simulink model "stm32f4_rtc_configure_demo"  (Simulink 7.3)
settings: Solver=FixedStepDiscrete  SolverMode=SingleTasking  StartTime=0.0  StopTime=10.0  RelTol=1e-3
PreLoadFcn:
  | waijung.modelPreload; % Required for working with Waijung Blockset. Do not remove.
undefined symbols (not defined in the file): HSEOSC, Link, LQFP176, ST, STM32F417IG
libraries: simulink x54, amg_high_precision_rtc x5, stm32f4_io_lib x2, stm32f4_device_config_lib x1
(part 2 of 3)

== system stm32f4_rtc_configure_demo/Display Date/Time/Display Second ==
  In1 : Inport
  In2 : Inport  Port=2
  In3 : Inport  Port=3
  Data Type Conversion : DataTypeConversion  OutDataTypeMode=uint8  OutDataType=fixdt(1, 16)  OutScaling=2^0  OutDataTypeStr=uint8
  Logical Operator : Logic  Inputs=3  AllPortsSameDT=off  OutDataTypeMode=boolean  LogicDataType=fixdt(0, 8)  OutDataTypeStr=boolean
  Switch : Switch  Criteria=u2 ~= 0  OutDataType=fixdt(1, 16)  OutScaling=2^0
  Volatile Data Storage Read : S-Function  FunctionName=waijung_vdata_read  Parameters=storagename,varname,sampletime,sampletimestr,blockid,storagetype,storagetypestr  EnableBusSupport=off  mask(waijung_vdata_read){storagename=str_blank2, varname=CharacterLCDSetupVolatileDataStorage7_str_blank2, sampletime=inf, sampletimestr=0.01, blockid=DisplayDateTimeDisplaySecondVolatileDataStorageRead, storagetype=string, storagetypestr=uint32_t}
      mask prompts: storagename "Storage Name"; varname "Variable name"; sampletime "Sample time (sec)"; sampletimestr "Compiled sample time (sec) in string"; storagetype "Data type"; storagetypestr "Data type string"
      mask help: This block implements read data from a buffer.
      mask init:
      | waijung_vdata_read_callback('init');
      mask Help: web(fullfile(waijungdocroot,'waijung_vdata_read.htm'))
      mask StyleString: popup(str_date|str_month|str_year|str_hour|str_minute|str_second|str_blank2|LCD_Buffer),edit,edit,edit,edit,edit,edit
      mask CallbackString: waijung_vdata_read_callback('storagename');|waijung_vdata_read_callback('varname');|waijung_vdata_read_callback('sampletime');|waijung_vdata_read_callback('sampletimestr');|waijung_vdata_read_callback('blockid');|waijung_vdata_read_callback('storagetype');|
      mask Display: text(0.05, 0.5, 'Buffer: str_blank2','ver','middle','hor','left');port_label('output',1,'D1(string)')
  Volatile Data Storage Read1 : S-Function  FunctionName=waijung_vdata_read  Parameters=storagename,varname,sampletime,sampletimestr,blockid,storagetype,storagetypestr  EnableBusSupport=off  mask(waijung_vdata_read){storagename=str_second, varname=CharacterLCDSetupVolatileDataStorage6_str_second, sampletime=inf, sampletimestr=0.01, blockid=DisplayDateTimeDisplaySecondVolatileDataStorageRead1, storagetype=string, storagetypestr=uint32_t}
      mask prompts: storagename "Storage Name"; varname "Variable name"; sampletime "Sample time (sec)"; sampletimestr "Compiled sample time (sec) in string"; storagetype "Data type"; storagetypestr "Data type string"
      mask help: This block implements read data from a buffer.
      mask init:
      | waijung_vdata_read_callback('init');
      mask Help: web(fullfile(waijungdocroot,'waijung_vdata_read.htm'))
      mask StyleString: popup(str_date|str_month|str_year|str_hour|str_minute|str_second|str_blank2|LCD_Buffer),edit,edit,edit,edit,edit,edit
      mask CallbackString: waijung_vdata_read_callback('storagename');|waijung_vdata_read_callback('varname');|waijung_vdata_read_callback('sampletime');|waijung_vdata_read_callback('sampletimestr');|waijung_vdata_read_callback('blockid');|waijung_vdata_read_callback('storagetype');|
      mask Display: text(0.05, 0.5, 'Buffer: str_second','ver','middle','hor','left');port_label('output',1,'D1(string)')
  Out1 : Outport
  wires:
  In3/1 -> Logical Operator/3
  Switch/1 -> Out1/1
  In2/1 -> Logical Operator/2
  In1/1 -> Logical Operator/1
  Volatile Data Storage Read1/1 -> Switch/3
  Volatile Data Storage Read/1 -> Switch/1
  Logical Operator/1 -> Data Type Conversion/1
  Data Type Conversion/1 -> Switch/2

== system stm32f4_rtc_configure_demo/Display Date/Time/Display Year ==
  In1 : Inport
  In2 : Inport  Port=2
  In3 : Inport  Port=3
  Data Type Conversion : DataTypeConversion  OutDataTypeMode=uint8  OutDataType=fixdt(1, 16)  OutScaling=2^0  OutDataTypeStr=uint8
  Logical Operator : Logic  Inputs=3  AllPortsSameDT=off  OutDataTypeMode=boolean  LogicDataType=fixdt(0, 8)  OutDataTypeStr=boolean
  Switch : Switch  Criteria=u2 ~= 0  OutDataType=fixdt(1, 16)  OutScaling=2^0
  Volatile Data Storage Read : S-Function  FunctionName=waijung_vdata_read  Parameters=storagename,varname,sampletime,sampletimestr,blockid,storagetype,storagetypestr  EnableBusSupport=off  mask(waijung_vdata_read){storagename=str_blank2, varname=CharacterLCDSetupVolatileDataStorage7_str_blank2, sampletime=inf, sampletimestr=0.01, blockid=DisplayDateTimeDisplayYearVolatileDataStorageRead, storagetype=string, storagetypestr=uint32_t}
      mask prompts: storagename "Storage Name"; varname "Variable name"; sampletime "Sample time (sec)"; sampletimestr "Compiled sample time (sec) in string"; storagetype "Data type"; storagetypestr "Data type string"
      mask help: This block implements read data from a buffer.
      mask init:
      | waijung_vdata_read_callback('init');
      mask Help: web(fullfile(waijungdocroot,'waijung_vdata_read.htm'))
      mask StyleString: popup(str_date|str_month|str_year|str_hour|str_minute|str_second|str_blank2|LCD_Buffer),edit,edit,edit,edit,edit,edit
      mask CallbackString: waijung_vdata_read_callback('storagename');|waijung_vdata_read_callback('varname');|waijung_vdata_read_callback('sampletime');|waijung_vdata_read_callback('sampletimestr');|waijung_vdata_read_callback('blockid');|waijung_vdata_read_callback('storagetype');|
      mask Display: text(0.05, 0.5, 'Buffer: str_blank2','ver','middle','hor','left');port_label('output',1,'D1(string)')
  Volatile Data Storage Read1 : S-Function  FunctionName=waijung_vdata_read  Parameters=storagename,varname,sampletime,sampletimestr,blockid,storagetype,storagetypestr  EnableBusSupport=off  mask(waijung_vdata_read){storagename=str_year, varname=CharacterLCDSetupVolatileDataStorage3_str_year, sampletime=inf, sampletimestr=0.01, blockid=DisplayDateTimeDisplayYearVolatileDataStorageRead1, storagetype=string, storagetypestr=uint32_t}
      mask prompts: storagename "Storage Name"; varname "Variable name"; sampletime "Sample time (sec)"; sampletimestr "Compiled sample time (sec) in string"; storagetype "Data type"; storagetypestr "Data type string"
      mask help: This block implements read data from a buffer.
      mask init:
      | waijung_vdata_read_callback('init');
      mask Help: web(fullfile(waijungdocroot,'waijung_vdata_read.htm'))
      mask StyleString: popup(str_date|str_month|str_year|str_hour|str_minute|str_second|str_blank2|LCD_Buffer),edit,edit,edit,edit,edit,edit
      mask CallbackString: waijung_vdata_read_callback('storagename');|waijung_vdata_read_callback('varname');|waijung_vdata_read_callback('sampletime');|waijung_vdata_read_callback('sampletimestr');|waijung_vdata_read_callback('blockid');|waijung_vdata_read_callback('storagetype');|
      mask Display: text(0.05, 0.5, 'Buffer: str_year','ver','middle','hor','left');port_label('output',1,'D1(string)')
  Out1 : Outport
  wires:
  Data Type Conversion/1 -> Switch/2
  Logical Operator/1 -> Data Type Conversion/1
  Volatile Data Storage Read/1 -> Switch/1
  Volatile Data Storage Read1/1 -> Switch/3
  In1/1 -> Logical Operator/1
  In2/1 -> Logical Operator/2
  Switch/1 -> Out1/1
  In3/1 -> Logical Operator/3

== system stm32f4_rtc_configure_demo/Display Date/Time/Get Date as String ==
  Printf1 : S-Function  FunctionName=waijung_printf  Parameters=storagename,printfformat,formatcode,varname,sampletime,sampletimestr,blockid  EnableBusSupport=off  mask(waijung_printf){storagename=str_date, printfformat=%2u/, formatcode=u, varname=CharacterLCDSetupVolatileDataStorage1_str_date, sampletime=-1, sampletimestr=0.01, blockid=DisplayDateTimeGetDateasStringPrintf1}
      mask prompts: storagename "Storage Name"; printfformat "Printf format"; formatcode "Printf format code"; varname "Variable name"; sampletime "Sample time (sec)"; sampletimestr "Compiled sample time (sec) in string"
      mask help: This block implements printf command.
      mask init:
      | waijung_printf_callback('init');
      mask Help: web(fullfile(waijungdocroot,'waijung_printf.htm'))
      mask StyleString: popup(str_date|str_month|str_year|str_hour|str_minute|str_second|str_blank2|LCD_Buffer),edit,edit,edit,edit,edit,edit
      mask CallbackString: waijung_printf_callback('storagename');|waijung_printf_callback('printfformat');|waijung_printf_callback('formatcode');|waijung_printf_callback('varname');|waijung_printf_callback('sampletime');|waijung_printf_callback('sampletimestr');|waijung_printf_callback('blockid');
      mask Display: text(0.95, 0.5, 'Buffer: str_date\nTs (sec): 0.01','ver','middle','hor','right');port_label('input',1,'D1(%u)');
  Printf2 : S-Function  FunctionName=waijung_printf  Parameters=storagename,printfformat,formatcode,varname,sampletime,sampletimestr,blockid  EnableBusSupport=off  mask(waijung_printf){storagename=str_month, printfformat=%2u/, formatcode=u, varname=CharacterLCDSetupVolatileDataStorage2_str_month, sampletime=-1, sampletimestr=0.01, blockid=DisplayDateTimeGetDateasStringPrintf2}
      mask prompts: storagename "Storage Name"; printfformat "Printf format"; formatcode "Printf format code"; varname "Variable name"; sampletime "Sample time (sec)"; sampletimestr "Compiled sample time (sec) in string"
      mask help: This block implements printf command.
      mask init:
      | waijung_printf_callback('init');
      mask Help: web(fullfile(waijungdocroot,'waijung_printf.htm'))
      mask StyleString: popup(str_date|str_month|str_year|str_hour|str_minute|str_second|str_blank2|LCD_Buffer),edit,edit,edit,edit,edit,edit
      mask CallbackString: waijung_printf_callback('storagename');|waijung_printf_callback('printfformat');|waijung_printf_callback('formatcode');|waijung_printf_callback('varname');|waijung_printf_callback('sampletime');|waijung_printf_callback('sampletimestr');|waijung_printf_callback('blockid');
      mask Display: text(0.95, 0.5, 'Buffer: str_month\nTs (sec): 0.01','ver','middle','hor','right');port_label('input',1,'D1(%u)');
  Printf3 : S-Function  FunctionName=waijung_printf  Parameters=storagename,printfformat,formatcode,varname,sampletime,sampletimestr,blockid  EnableBusSupport=off  mask(waijung_printf){storagename=str_year, printfformat=%2u, formatcode=u, varname=CharacterLCDSetupVolatileDataStorage3_str_year, sampletime=-1, sampletimestr=0.01, blockid=DisplayDateTimeGetDateasStringPrintf3}
      mask prompts: storagename "Storage Name"; printfformat "Printf format"; formatcode "Printf format code"; varname "Variable name"; sampletime "Sample time (sec)"; sampletimestr "Compiled sample time (sec) in string"
      mask help: This block implements printf command.
      mask init:
      | waijung_printf_callback('init');
      mask Help: web(fullfile(waijungdocroot,'waijung_printf.htm'))
      mask StyleString: popup(str_date|str_month|str_year|str_hour|str_minute|str_second|str_blank2|LCD_Buffer),edit,edit,edit,edit,edit,edit
      mask CallbackString: waijung_printf_callback('storagename');|waijung_printf_callback('printfformat');|waijung_printf_callback('formatcode');|waijung_printf_callback('varname');|waijung_printf_callback('sampletime');|waijung_printf_callback('sampletimestr');|waijung_printf_callback('blockid');
      mask Display: text(0.95, 0.5, 'Buffer: str_year\nTs (sec): 0.01','ver','middle','hor','right');port_label('input',1,'D1(%u)');
  RTC Date Read : S-Function  FunctionName=stm32f4_rtc  Parameters=inputtypearray,outputtypearray,confstr,sampletime,sampletimestr,blockid  EnableBusSupport=off  mask(stm32f4_rtc){configuration=DateRead, clocksource=LSE (32.768kHz), dataformat=BIN, hourformat=HourFormat_24, inputtypearray=[0], outputtypearray=[4 3 3 3 3], confstr=["DateRead","LSE (32.768kHz)","BIN","HourFormat_24"], sampletime=0.01, sampletimestr=0.01, blockid=DisplayDateTimeGetDateasStringRTCDateRead}
      mask prompts: clocksource "Clock source"; dataformat "Format"; hourformat "Hour format"; inputtypearray "Input type array"; outputtypearray "Output type array"; confstr "Configuration string"; sampletime "Sample time (sec)"; sampletimestr "Compiled sample time (sec) in string"
      mask init:
      | stm32f4_rtc_callback('init');
      mask Help: web(fullfile(waijungdocroot,'stm32f4_rtc_setup.htm'), '-browser')
      mask StyleString: popup(Setup|DateRead|TimeRead|DateWrite|TimeWrite),popup(LSE (32.768kHz)|LSI),popup(BCD|BIN),popup(HourFormat_24|HourFormat_12),edit,edit,edit,edit,edit,edit
      mask CallbackString: stm32f4_rtc_callback('configuration');||stm32f4_rtc_callback('dataformat');||||stm32f4_rtc_callback('confstr');|stm32f4_rtc_callback('sampletime');|stm32f4_rtc_callback('sampletimestr');|stm32f4_rtc_callback('blockid');
      mask Display: text(0.05, 0.5, 'Module: RTC (DateRead)\nFormat: BIN\nTs (sec): 0.01','ver','middle','hor','left');port_label('output', 1,'Day');port_label('output', 2,'Date');port_label('output', 3,'Month');port_label('output', 4,'Year');
  Terminator : Terminator
  wires:
  RTC Date Read/2 -> Printf1/1
  RTC Date Read/4 -> Printf3/1
  RTC Date Read/3 -> Printf2/1
  RTC Date Read/1 -> Terminator/1

== system stm32f4_rtc_configure_demo/Display Date/Time/Get Time as String ==
  Printf4 : S-Function  FunctionName=waijung_printf  Parameters=storagename,printfformat,formatcode,varname,sampletime,sampletimestr,blockid  EnableBusSupport=off  mask(waijung_printf){storagename=str_hour, printfformat=%2u:, formatcode=u, varname=CharacterLCDSetupVolatileDataStorage4_str_hour, sampletime=-1, sampletimestr=0.01, blockid=DisplayDateTimeGetTimeasStringPrintf4}
      mask prompts: storagename "Storage Name"; printfformat "Printf format"; formatcode "Printf format code"; varname "Variable name"; sampletime "Sample time (sec)"; sampletimestr "Compiled sample time (sec) in string"
      mask help: This block implements printf command.
      mask init:
      | waijung_printf_callback('init');
      mask Help: web(fullfile(waijungdocroot,'waijung_printf.htm'))
      mask StyleString: popup(str_date|str_month|str_year|str_hour|str_minute|str_second|str_blank2|LCD_Buffer),edit,edit,edit,edit,edit,edit
      mask CallbackString: waijung_printf_callback('storagename');|waijung_printf_callback('printfformat');|waijung_printf_callback('formatcode');|waijung_printf_callback('varname');|waijung_printf_callback('sampletime');|waijung_printf_callback('sampletimestr');|waijung_printf_callback('blockid');
      mask Display: text(0.95, 0.5, 'Buffer: str_hour\nTs (sec): 0.01','ver','middle','hor','right');port_label('input',1,'D1(%u)');
  Printf5 : S-Function  FunctionName=waijung_printf  Parameters=storagename,printfformat,formatcode,varname,sampletime,sampletimestr,blockid  EnableBusSupport=off  mask(waijung_printf){storagename=str_minute, printfformat=%2u:, formatcode=u, varname=CharacterLCDSetupVolatileDataStorage5_str_minute, sampletime=-1, sampletimestr=0.01, blockid=DisplayDateTimeGetTimeasStringPrintf5}
      mask prompts: storagename "Storage Name"; printfformat "Printf format"; formatcode "Printf format code"; varname "Variable name"; sampletime "Sample time (sec)"; sampletimestr "Compiled sample time (sec) in string"
      mask help: This block implements printf command.
      mask init:
      | waijung_printf_callback('init');
      mask Help: web(fullfile(waijungdocroot,'waijung_printf.htm'))
      mask StyleString: popup(str_date|str_month|str_year|str_hour|str_minute|str_second|str_blank2|LCD_Buffer),edit,edit,edit,edit,edit,edit
      mask CallbackString: waijung_printf_callback('storagename');|waijung_printf_callback('printfformat');|waijung_printf_callback('formatcode');|waijung_printf_callback('varname');|waijung_printf_callback('sampletime');|waijung_printf_callback('sampletimestr');|waijung_printf_callback('blockid');
      mask Display: text(0.95, 0.5, 'Buffer: str_minute\nTs (sec): 0.01','ver','middle','hor','right');port_label('input',1,'D1(%u)');
  Printf6 : S-Function  FunctionName=waijung_printf  Parameters=storagename,printfformat,formatcode,varname,sampletime,sampletimestr,blockid  EnableBusSupport=off  mask(waijung_printf){storagename=str_second, printfformat=%2u, formatcode=u, varname=CharacterLCDSetupVolatileDataStorage6_str_second, sampletime=-1, sampletimestr=0.01, blockid=DisplayDateTimeGetTimeasStringPrintf6}
      mask prompts: storagename "Storage Name"; printfformat "Printf format"; formatcode "Printf format code"; varname "Variable name"; sampletime "Sample time (sec)"; sampletimestr "Compiled sample time (sec) in string"
      mask help: This block implements printf command.
      mask init:
      | waijung_printf_callback('init');
      mask Help: web(fullfile(waijungdocroot,'waijung_printf.htm'))
      mask StyleString: popup(str_date|str_month|str_year|str_hour|str_minute|str_second|str_blank2|LCD_Buffer),edit,edit,edit,edit,edit,edit
      mask CallbackString: waijung_printf_callback('storagename');|waijung_printf_callback('printfformat');|waijung_printf_callback('formatcode');|waijung_printf_callback('varname');|waijung_printf_callback('sampletime');|waijung_printf_callback('sampletimestr');|waijung_printf_callback('blockid');
      mask Display: text(0.95, 0.5, 'Buffer: str_second\nTs (sec): 0.01','ver','middle','hor','right');port_label('input',1,'D1(%u)');
  RTC Time Read : S-Function  FunctionName=stm32f4_rtc  Parameters=inputtypearray,outputtypearray,confstr,sampletime,sampletimestr,blockid  EnableBusSupport=off  mask(stm32f4_rtc){configuration=TimeRead, clocksource=LSE (32.768kHz), dataformat=BIN, hourformat=HourFormat_24, inputtypearray=[0], outputtypearray=[3 3 3 3], confstr=["TimeRead","LSE (32.768kHz)","BIN","HourFormat_24"], sampletime=0.01, sampletimestr=0.01, blockid=DisplayDateTimeGetTimeasStringRTCTimeRead}
      mask prompts: clocksource "Clock source"; dataformat "Format"; hourformat "Hour format"; inputtypearray "Input type array"; outputtypearray "Output type array"; confstr "Configuration string"; sampletime "Sample time (sec)"; sampletimestr "Compiled sample time (sec) in string"
      mask init:
      | stm32f4_rtc_callback('init');
      mask Help: web(fullfile(waijungdocroot,'stm32f4_rtc_setup.htm'), '-browser')
      mask StyleString: popup(Setup|DateRead|TimeRead|DateWrite|TimeWrite),popup(LSE (32.768kHz)|LSI),popup(BCD|BIN),popup(HourFormat_24|HourFormat_12),edit,edit,edit,edit,edit,edit
      mask CallbackString: stm32f4_rtc_callback('configuration');||stm32f4_rtc_callback('dataformat');||||stm32f4_rtc_callback('confstr');|stm32f4_rtc_callback('sampletime');|stm32f4_rtc_callback('sampletimestr');|stm32f4_rtc_callback('blockid');
      mask Display: text(0.05, 0.5, 'Module: RTC (TimeRead)\nFormat: BIN\nTs (sec): 0.01','ver','middle','hor','left');port_label('output', 1,'Hour');port_label('output', 2,'Minute');port_label('output', 3,'Second');
  wires:
  RTC Time Read/3 -> Printf6/1
  RTC Time Read/2 -> Printf5/1
  RTC Time Read/1 -> Printf4/1

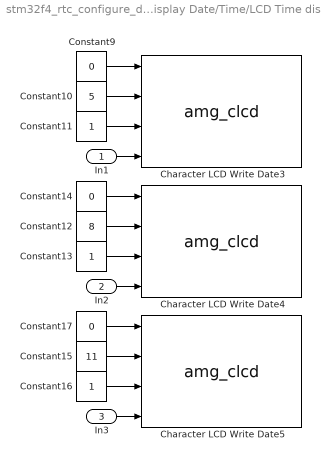
== system stm32f4_rtc_configure_demo/Display Date/Time/LCD Time display ==
  In1 : Inport
  In2 : Inport  Port=2
  In3 : Inport  Port=3
  Character LCD Write Date3 : S-Function  FunctionName=amg_clcd  Parameters=module,configuration,inputtypearray,outputtypearray,confstr,sampletime,sampletimestr,blockid  EnableBusSupport=off  mask(amg_clcd){configuration=Transaction, module=1, model=amg CLCD Std, interface=4-bits, linecount=4, columncount=20, gpiotype=Push-pull, controlport=E, control_rs=15, control_rw=13, control_en=11, dataport=A, data0=7, data1=5, data2=3, data3=1, usestringbuffer=off, stringbuffer=<empty>, varname=, inputtypearray=[4 -1 -1 -1 -1], outputtypearray=[0], confstr=["4","4","20","PP","E","15","11","13","","A","","","","","7","5","3","1","0","","1","0","0","0","1","0","0","0","0","stm32f4"], sampletime=-1, sampletimestr=0.01, blockid=DisplayDateTimeLCDTimedisplayCharacterLCDWriteDate3}
      mask prompts: model "LCD model:"; linecount "Number of lines:"; columncount "Number of columns:"; gpiotype "GPIO Output type:"; controlport "GPIO control port:"; control_rs "GPIO control pin, RS:"; control_rw "GPIO control pin, RW:"; control_en "GPIO control pin, EN:"; dataport "GPIO data D[7:4] port"; data0 "GPIO data pin, D4:"; data1 "GPIO data pin, D5:"; data2 "GPIO data pin, D6:"; data3 "GPIO data pin, D7:"; usestringbuffer "Use string buffer"; stringbuffer "String buffer"; varname "Variable name"; inputtypearray "Input type array"; outputtypearray "Output type array"; confstr "Configuration string"; sampletime "Sample time (sec)"; sampletimestr "Compiled sample time (sec) in string"
      mask help:
      | Note for cmd:
      | 1 - Clear LCD Line before write.
      | 0 or otherwise - Write into LCD Line with existing data.
      mask init:
      | amg_clcd_callback('init');
      mask Help: web(fullfile(waijungdocroot,'amg_clcd_write.htm'), '-browser')
      mask StyleString: popup(Setup|Transaction),popup(1|2|3|4),popup(amg CLCD Std),popup(4-bits),edit,edit,popup(Push-pull|Open-drain),popup(A|B|C|D|E|F|G|H|I),popup(0|1|2|3|4|5|6|7|8|9|10|11|12|13|14|15),popup(0|1|2|3|4|5|6|7|8|9|10|11|12|13|14|15),popup(0|1|2|3|4|5|6|7|8|9|10|11|12|13|14|15),popup(A|B|C|D|E|F|G|H|I),popup(0|1|2|3|4|5|6|7|8|9|10|11|12|13|14|15),popup(0|1|2|3|4|5|6|7|8|9|10|11|12|13|14|15),popup(0|1|2|3|4|5|6|7|8|9|10|11|12|13|14|15),popup(0|1|2|3|4|5|6|7|8|9|10|11|12|13|14|15),checkbox,popup(str_date|str_month|str_year|str_hour|str_minute|str_second|str_blank2|LCD_Buffer|<empty>),edit,edit,edit,edit,edit,edit,edit
      mask CallbackString: amg_clcd_callback('configuration');||||||||||||||||amg_clcd_callback('usestringbuffer');||amg_clcd_callback('varname');|||amg_clcd_callback('confstr');|amg_clcd_callback('sampletime');|amg_clcd_callback('sampletimestr');|amg_clcd_callback('blockid');
      mask Display: text(0.5, 0.5, 'Module: CLCD1 (Write)\nTs (sec): 0.01','ver','middle','hor','center');port_label('input', 1,'cmd');port_label('input', 2,'xpos');port_label('input', 3,'ypos');port_label('input', 4,'str');
  Character LCD Write Date4 : S-Function  FunctionName=amg_clcd  Parameters=module,configuration,inputtypearray,outputtypearray,confstr,sampletime,sampletimestr,blockid  EnableBusSupport=off  mask(amg_clcd){configuration=Transaction, module=1, model=amg CLCD Std, interface=4-bits, linecount=4, columncount=20, gpiotype=Push-pull, controlport=E, control_rs=15, control_rw=13, control_en=11, dataport=A, data0=7, data1=5, data2=3, data3=1, usestringbuffer=off, stringbuffer=<empty>, varname=, inputtypearray=[4 -1 -1 -1 -1], outputtypearray=[0], confstr=["4","4","20","PP","E","15","11","13","","A","","","","","7","5","3","1","0","","1","0","0","0","1","0","0","0","0","stm32f4"], sampletime=-1, sampletimestr=0.01, blockid=DisplayDateTimeLCDTimedisplayCharacterLCDWriteDate4}
      mask prompts: model "LCD model:"; linecount "Number of lines:"; columncount "Number of columns:"; gpiotype "GPIO Output type:"; controlport "GPIO control port:"; control_rs "GPIO control pin, RS:"; control_rw "GPIO control pin, RW:"; control_en "GPIO control pin, EN:"; dataport "GPIO data D[7:4] port"; data0 "GPIO data pin, D4:"; data1 "GPIO data pin, D5:"; data2 "GPIO data pin, D6:"; data3 "GPIO data pin, D7:"; usestringbuffer "Use string buffer"; stringbuffer "String buffer"; varname "Variable name"; inputtypearray "Input type array"; outputtypearray "Output type array"; confstr "Configuration string"; sampletime "Sample time (sec)"; sampletimestr "Compiled sample time (sec) in string"
      mask help:
      | Note for cmd:
      | 1 - Clear LCD Line before write.
      | 0 or otherwise - Write into LCD Line with existing data.
      mask init:
      | amg_clcd_callback('init');
      mask Help: web(fullfile(waijungdocroot,'amg_clcd_write.htm'), '-browser')
      mask StyleString: popup(Setup|Transaction),popup(1|2|3|4),popup(amg CLCD Std),popup(4-bits),edit,edit,popup(Push-pull|Open-drain),popup(A|B|C|D|E|F|G|H|I),popup(0|1|2|3|4|5|6|7|8|9|10|11|12|13|14|15),popup(0|1|2|3|4|5|6|7|8|9|10|11|12|13|14|15),popup(0|1|2|3|4|5|6|7|8|9|10|11|12|13|14|15),popup(A|B|C|D|E|F|G|H|I),popup(0|1|2|3|4|5|6|7|8|9|10|11|12|13|14|15),popup(0|1|2|3|4|5|6|7|8|9|10|11|12|13|14|15),popup(0|1|2|3|4|5|6|7|8|9|10|11|12|13|14|15),popup(0|1|2|3|4|5|6|7|8|9|10|11|12|13|14|15),checkbox,popup(str_date|str_month|str_year|str_hour|str_minute|str_second|str_blank2|LCD_Buffer|<empty>),edit,edit,edit,edit,edit,edit,edit
      mask CallbackString: amg_clcd_callback('configuration');||||||||||||||||amg_clcd_callback('usestringbuffer');||amg_clcd_callback('varname');|||amg_clcd_callback('confstr');|amg_clcd_callback('sampletime');|amg_clcd_callback('sampletimestr');|amg_clcd_callback('blockid');
      mask Display: text(0.5, 0.5, 'Module: CLCD1 (Write)\nTs (sec): 0.01','ver','middle','hor','center');port_label('input', 1,'cmd');port_label('input', 2,'xpos');port_label('input', 3,'ypos');port_label('input', 4,'str');
  Character LCD Write Date5 : S-Function  FunctionName=amg_clcd  Parameters=module,configuration,inputtypearray,outputtypearray,confstr,sampletime,sampletimestr,blockid  EnableBusSupport=off  mask(amg_clcd){configuration=Transaction, module=1, model=amg CLCD Std, interface=4-bits, linecount=4, columncount=20, gpiotype=Push-pull, controlport=E, control_rs=15, control_rw=13, control_en=11, dataport=A, data0=7, data1=5, data2=3, data3=1, usestringbuffer=off, stringbuffer=<empty>, varname=, inputtypearray=[4 -1 -1 -1 -1], outputtypearray=[0], confstr=["4","4","20","PP","E","15","11","13","","A","","","","","7","5","3","1","0","","1","0","0","0","1","0","0","0","0","stm32f4"], sampletime=-1, sampletimestr=0.01, blockid=DisplayDateTimeLCDTimedisplayCharacterLCDWriteDate5}
      mask prompts: model "LCD model:"; linecount "Number of lines:"; columncount "Number of columns:"; gpiotype "GPIO Output type:"; controlport "GPIO control port:"; control_rs "GPIO control pin, RS:"; control_rw "GPIO control pin, RW:"; control_en "GPIO control pin, EN:"; dataport "GPIO data D[7:4] port"; data0 "GPIO data pin, D4:"; data1 "GPIO data pin, D5:"; data2 "GPIO data pin, D6:"; data3 "GPIO data pin, D7:"; usestringbuffer "Use string buffer"; stringbuffer "String buffer"; varname "Variable name"; inputtypearray "Input type array"; outputtypearray "Output type array"; confstr "Configuration string"; sampletime "Sample time (sec)"; sampletimestr "Compiled sample time (sec) in string"
      mask help:
      | Note for cmd:
      | 1 - Clear LCD Line before write.
      | 0 or otherwise - Write into LCD Line with existing data.
      mask init:
      | amg_clcd_callback('init');
      mask Help: web(fullfile(waijungdocroot,'amg_clcd_write.htm'), '-browser')
      mask StyleString: popup(Setup|Transaction),popup(1|2|3|4),popup(amg CLCD Std),popup(4-bits),edit,edit,popup(Push-pull|Open-drain),popup(A|B|C|D|E|F|G|H|I),popup(0|1|2|3|4|5|6|7|8|9|10|11|12|13|14|15),popup(0|1|2|3|4|5|6|7|8|9|10|11|12|13|14|15),popup(0|1|2|3|4|5|6|7|8|9|10|11|12|13|14|15),popup(A|B|C|D|E|F|G|H|I),popup(0|1|2|3|4|5|6|7|8|9|10|11|12|13|14|15),popup(0|1|2|3|4|5|6|7|8|9|10|11|12|13|14|15),popup(0|1|2|3|4|5|6|7|8|9|10|11|12|13|14|15),popup(0|1|2|3|4|5|6|7|8|9|10|11|12|13|14|15),checkbox,popup(str_date|str_month|str_year|str_hour|str_minute|str_second|str_blank2|LCD_Buffer|<empty>),edit,edit,edit,edit,edit,edit,edit
      mask CallbackString: amg_clcd_callback('configuration');||||||||||||||||amg_clcd_callback('usestringbuffer');||amg_clcd_callback('varname');|||amg_clcd_callback('confstr');|amg_clcd_callback('sampletime');|amg_clcd_callback('sampletimestr');|amg_clcd_callback('blockid');
      mask Display: text(0.5, 0.5, 'Module: CLCD1 (Write)\nTs (sec): 0.01','ver','middle','hor','center');port_label('input', 1,'cmd');port_label('input', 2,'xpos');port_label('input', 3,'ypos');port_label('input', 4,'str');
  Constant10 : Constant  Value=5  OutDataTypeMode=uint8  OutDataType=fixdt(1, 16)  OutScaling=2^0  OutDataTypeStr=uint8
  Constant11 : Constant  OutDataTypeMode=uint8  OutDataType=fixdt(1, 16)  OutScaling=2^0  OutDataTypeStr=uint8
  Constant12 : Constant  Value=8  OutDataTypeMode=uint8  OutDataType=fixdt(1, 16)  OutScaling=2^0  OutDataTypeStr=uint8
  Constant13 : Constant  OutDataTypeMode=uint8  OutDataType=fixdt(1, 16)  OutScaling=2^0  OutDataTypeStr=uint8
  Constant14 : Constant  Value=0  OutDataTypeMode=uint8  OutDataType=fixdt(1, 16)  OutScaling=2^0  OutDataTypeStr=uint8
  Constant15 : Constant  Value=11  OutDataTypeMode=uint8  OutDataType=fixdt(1, 16)  OutScaling=2^0  OutDataTypeStr=uint8
  Constant16 : Constant  OutDataTypeMode=uint8  OutDataType=fixdt(1, 16)  OutScaling=2^0  OutDataTypeStr=uint8
  Constant17 : Constant  Value=0  OutDataTypeMode=uint8  OutDataType=fixdt(1, 16)  OutScaling=2^0  OutDataTypeStr=uint8
  Constant9 : Constant  Value=0  OutDataTypeMode=uint8  OutDataType=fixdt(1, 16)  OutScaling=2^0  OutDataTypeStr=uint8
  wires:
  Constant10/1 -> Character LCD Write Date3/2
  Constant11/1 -> Character LCD Write Date3/3
  Constant9/1 -> Character LCD Write Date3/1
  Constant12/1 -> Character LCD Write Date4/2
  Constant13/1 -> Character LCD Write Date4/3
  Constant14/1 -> Character LCD Write Date4/1
  Constant15/1 -> Character LCD Write Date5/2
  Constant16/1 -> Character LCD Write Date5/3
  Constant17/1 -> Character LCD Write Date5/1
  In1/1 -> Character LCD Write Date3/4
  In2/1 -> Character LCD Write Date4/4
  In3/1 -> Character LCD Write Date5/4

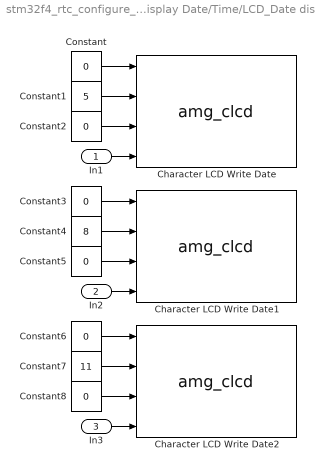
== system stm32f4_rtc_configure_demo/Display Date/Time/LCD_Date display ==
  In1 : Inport
  In2 : Inport  Port=2
  In3 : Inport  Port=3
  Character LCD Write Date : S-Function  FunctionName=amg_clcd  Parameters=module,configuration,inputtypearray,outputtypearray,confstr,sampletime,sampletimestr,blockid  EnableBusSupport=off  mask(amg_clcd){configuration=Transaction, module=1, model=amg CLCD Std, interface=4-bits, linecount=4, columncount=20, gpiotype=Push-pull, controlport=E, control_rs=15, control_rw=13, control_en=11, dataport=A, data0=7, data1=5, data2=3, data3=1, usestringbuffer=off, stringbuffer=<empty>, varname=, inputtypearray=[4 -1 -1 -1 -1], outputtypearray=[0], confstr=["4","4","20","PP","E","15","11","13","","A","","","","","7","5","3","1","0","","1","0","0","0","1","0","0","0","0","stm32f4"], sampletime=-1, sampletimestr=0.01, blockid=DisplayDateTimeLCD_DatedisplayCharacterLCDWriteDate}
      mask prompts: model "LCD model:"; linecount "Number of lines:"; columncount "Number of columns:"; gpiotype "GPIO Output type:"; controlport "GPIO control port:"; control_rs "GPIO control pin, RS:"; control_rw "GPIO control pin, RW:"; control_en "GPIO control pin, EN:"; dataport "GPIO data D[7:4] port"; data0 "GPIO data pin, D4:"; data1 "GPIO data pin, D5:"; data2 "GPIO data pin, D6:"; data3 "GPIO data pin, D7:"; usestringbuffer "Use string buffer"; stringbuffer "String buffer"; varname "Variable name"; inputtypearray "Input type array"; outputtypearray "Output type array"; confstr "Configuration string"; sampletime "Sample time (sec)"; sampletimestr "Compiled sample time (sec) in string"
      mask help:
      | Note for cmd:
      | 1 - Clear LCD Line before write.
      | 0 or otherwise - Write into LCD Line with existing data.
      mask init:
      | amg_clcd_callback('init');
      mask Help: web(fullfile(waijungdocroot,'amg_clcd_write.htm'), '-browser')
      mask StyleString: popup(Setup|Transaction),popup(1|2|3|4),popup(amg CLCD Std),popup(4-bits),edit,edit,popup(Push-pull|Open-drain),popup(A|B|C|D|E|F|G|H|I),popup(0|1|2|3|4|5|6|7|8|9|10|11|12|13|14|15),popup(0|1|2|3|4|5|6|7|8|9|10|11|12|13|14|15),popup(0|1|2|3|4|5|6|7|8|9|10|11|12|13|14|15),popup(A|B|C|D|E|F|G|H|I),popup(0|1|2|3|4|5|6|7|8|9|10|11|12|13|14|15),popup(0|1|2|3|4|5|6|7|8|9|10|11|12|13|14|15),popup(0|1|2|3|4|5|6|7|8|9|10|11|12|13|14|15),popup(0|1|2|3|4|5|6|7|8|9|10|11|12|13|14|15),checkbox,popup(str_date|str_month|str_year|str_hour|str_minute|str_second|str_blank2|LCD_Buffer|<empty>),edit,edit,edit,edit,edit,edit,edit
      mask CallbackString: amg_clcd_callback('configuration');||||||||||||||||amg_clcd_callback('usestringbuffer');||amg_clcd_callback('varname');|||amg_clcd_callback('confstr');|amg_clcd_callback('sampletime');|amg_clcd_callback('sampletimestr');|amg_clcd_callback('blockid');
      mask Display: text(0.5, 0.5, 'Module: CLCD1 (Write)\nTs (sec): 0.01','ver','middle','hor','center');port_label('input', 1,'cmd');port_label('input', 2,'xpos');port_label('input', 3,'ypos');port_label('input', 4,'str');
  Character LCD Write Date1 : S-Function  FunctionName=amg_clcd  Parameters=module,configuration,inputtypearray,outputtypearray,confstr,sampletime,sampletimestr,blockid  EnableBusSupport=off  mask(amg_clcd){configuration=Transaction, module=1, model=amg CLCD Std, interface=4-bits, linecount=4, columncount=20, gpiotype=Push-pull, controlport=E, control_rs=15, control_rw=13, control_en=11, dataport=A, data0=7, data1=5, data2=3, data3=1, usestringbuffer=off, stringbuffer=<empty>, varname=, inputtypearray=[4 -1 -1 -1 -1], outputtypearray=[0], confstr=["4","4","20","PP","E","15","11","13","","A","","","","","7","5","3","1","0","","1","0","0","0","1","0","0","0","0","stm32f4"], sampletime=-1, sampletimestr=0.01, blockid=DisplayDateTimeLCD_DatedisplayCharacterLCDWriteDate1}
      mask prompts: model "LCD model:"; linecount "Number of lines:"; columncount "Number of columns:"; gpiotype "GPIO Output type:"; controlport "GPIO control port:"; control_rs "GPIO control pin, RS:"; control_rw "GPIO control pin, RW:"; control_en "GPIO control pin, EN:"; dataport "GPIO data D[7:4] port"; data0 "GPIO data pin, D4:"; data1 "GPIO data pin, D5:"; data2 "GPIO data pin, D6:"; data3 "GPIO data pin, D7:"; usestringbuffer "Use string buffer"; stringbuffer "String buffer"; varname "Variable name"; inputtypearray "Input type array"; outputtypearray "Output type array"; confstr "Configuration string"; sampletime "Sample time (sec)"; sampletimestr "Compiled sample time (sec) in string"
      mask help:
      | Note for cmd:
      | 1 - Clear LCD Line before write.
      | 0 or otherwise - Write into LCD Line with existing data.
      mask init:
      | amg_clcd_callback('init');
      mask Help: web(fullfile(waijungdocroot,'amg_clcd_write.htm'), '-browser')
      mask StyleString: popup(Setup|Transaction),popup(1|2|3|4),popup(amg CLCD Std),popup(4-bits),edit,edit,popup(Push-pull|Open-drain),popup(A|B|C|D|E|F|G|H|I),popup(0|1|2|3|4|5|6|7|8|9|10|11|12|13|14|15),popup(0|1|2|3|4|5|6|7|8|9|10|11|12|13|14|15),popup(0|1|2|3|4|5|6|7|8|9|10|11|12|13|14|15),popup(A|B|C|D|E|F|G|H|I),popup(0|1|2|3|4|5|6|7|8|9|10|11|12|13|14|15),popup(0|1|2|3|4|5|6|7|8|9|10|11|12|13|14|15),popup(0|1|2|3|4|5|6|7|8|9|10|11|12|13|14|15),popup(0|1|2|3|4|5|6|7|8|9|10|11|12|13|14|15),checkbox,popup(str_date|str_month|str_year|str_hour|str_minute|str_second|str_blank2|LCD_Buffer|<empty>),edit,edit,edit,edit,edit,edit,edit
      mask CallbackString: amg_clcd_callback('configuration');||||||||||||||||amg_clcd_callback('usestringbuffer');||amg_clcd_callback('varname');|||amg_clcd_callback('confstr');|amg_clcd_callback('sampletime');|amg_clcd_callback('sampletimestr');|amg_clcd_callback('blockid');
      mask Display: text(0.5, 0.5, 'Module: CLCD1 (Write)\nTs (sec): 0.01','ver','middle','hor','center');port_label('input', 1,'cmd');port_label('input', 2,'xpos');port_label('input', 3,'ypos');port_label('input', 4,'str');
  Character LCD Write Date2 : S-Function  FunctionName=amg_clcd  Parameters=module,configuration,inputtypearray,outputtypearray,confstr,sampletime,sampletimestr,blockid  EnableBusSupport=off  mask(amg_clcd){configuration=Transaction, module=1, model=amg CLCD Std, interface=4-bits, linecount=4, columncount=20, gpiotype=Push-pull, controlport=E, control_rs=15, control_rw=13, control_en=11, dataport=A, data0=7, data1=5, data2=3, data3=1, usestringbuffer=off, stringbuffer=<empty>, varname=, inputtypearray=[4 -1 -1 -1 -1], outputtypearray=[0], confstr=["4","4","20","PP","E","15","11","13","","A","","","","","7","5","3","1","0","","1","0","0","0","1","0","0","0","0","stm32f4"], sampletime=-1, sampletimestr=0.01, blockid=DisplayDateTimeLCD_DatedisplayCharacterLCDWriteDate2}
      mask prompts: model "LCD model:"; linecount "Number of lines:"; columncount "Number of columns:"; gpiotype "GPIO Output type:"; controlport "GPIO control port:"; control_rs "GPIO control pin, RS:"; control_rw "GPIO control pin, RW:"; control_en "GPIO control pin, EN:"; dataport "GPIO data D[7:4] port"; data0 "GPIO data pin, D4:"; data1 "GPIO data pin, D5:"; data2 "GPIO data pin, D6:"; data3 "GPIO data pin, D7:"; usestringbuffer "Use string buffer"; stringbuffer "String buffer"; varname "Variable name"; inputtypearray "Input type array"; outputtypearray "Output type array"; confstr "Configuration string"; sampletime "Sample time (sec)"; sampletimestr "Compiled sample time (sec) in string"
      mask help:
      | Note for cmd:
      | 1 - Clear LCD Line before write.
      | 0 or otherwise - Write into LCD Line with existing data.
      mask init:
      | amg_clcd_callback('init');
      mask Help: web(fullfile(waijungdocroot,'amg_clcd_write.htm'), '-browser')
      mask StyleString: popup(Setup|Transaction),popup(1|2|3|4),popup(amg CLCD Std),popup(4-bits),edit,edit,popup(Push-pull|Open-drain),popup(A|B|C|D|E|F|G|H|I),popup(0|1|2|3|4|5|6|7|8|9|10|11|12|13|14|15),popup(0|1|2|3|4|5|6|7|8|9|10|11|12|13|14|15),popup(0|1|2|3|4|5|6|7|8|9|10|11|12|13|14|15),popup(A|B|C|D|E|F|G|H|I),popup(0|1|2|3|4|5|6|7|8|9|10|11|12|13|14|15),popup(0|1|2|3|4|5|6|7|8|9|10|11|12|13|14|15),popup(0|1|2|3|4|5|6|7|8|9|10|11|12|13|14|15),popup(0|1|2|3|4|5|6|7|8|9|10|11|12|13|14|15),checkbox,popup(str_date|str_month|str_year|str_hour|str_minute|str_second|str_blank2|LCD_Buffer|<empty>),edit,edit,edit,edit,edit,edit,edit
      mask CallbackString: amg_clcd_callback('configuration');||||||||||||||||amg_clcd_callback('usestringbuffer');||amg_clcd_callback('varname');|||amg_clcd_callback('confstr');|amg_clcd_callback('sampletime');|amg_clcd_callback('sampletimestr');|amg_clcd_callback('blockid');
      mask Display: text(0.5, 0.5, 'Module: CLCD1 (Write)\nTs (sec): 0.01','ver','middle','hor','center');port_label('input', 1,'cmd');port_label('input', 2,'xpos');port_label('input', 3,'ypos');port_label('input', 4,'str');
  Constant{,2..3,5..6,8} (6 alike) : Constant  Value=0  OutDataTypeMode=uint8  OutDataType=fixdt(1, 16)  OutScaling=2^0  OutDataTypeStr=uint8
  Constant1 : Constant  Value=5  OutDataTypeMode=uint8  OutDataType=fixdt(1, 16)  OutScaling=2^0  OutDataTypeStr=uint8
  Constant4 : Constant  Value=8  OutDataTypeMode=uint8  OutDataType=fixdt(1, 16)  OutScaling=2^0  OutDataTypeStr=uint8
  Constant7 : Constant  Value=11  OutDataTypeMode=uint8  OutDataType=fixdt(1, 16)  OutScaling=2^0  OutDataTypeStr=uint8
  wires:
  Constant/1 -> Character LCD Write Date/1
  Constant1/1 -> Character LCD Write Date/2
  Constant2/1 -> Character LCD Write Date/3
  Constant3/1 -> Character LCD Write Date1/1
  Constant4/1 -> Character LCD Write Date1/2
  Constant5/1 -> Character LCD Write Date1/3
  Constant7/1 -> Character LCD Write Date2/2
  Constant8/1 -> Character LCD Write Date2/3
  Constant6/1 -> Character LCD Write Date2/1
  In1/1 -> Character LCD Write Date/4
  In2/1 -> Character LCD Write Date1/4
  In3/1 -> Character LCD Write Date2/4

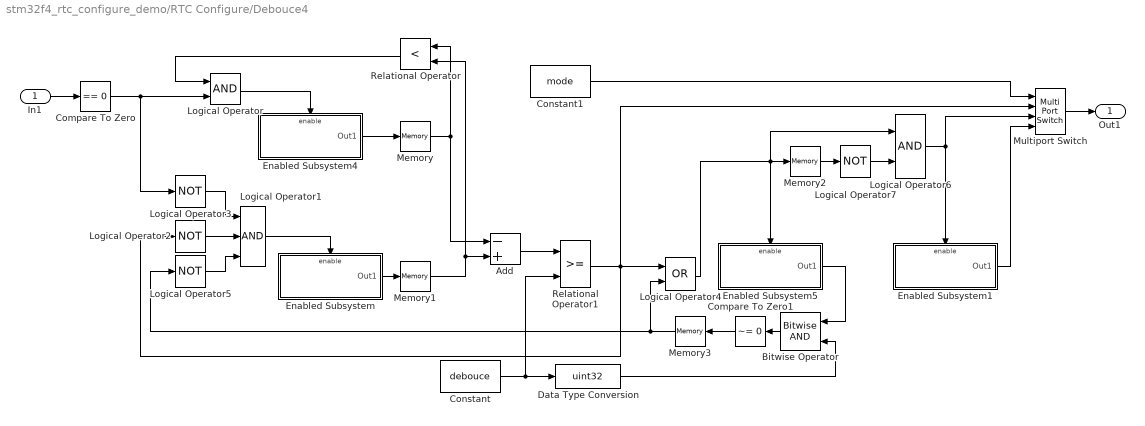
== system stm32f4_rtc_configure_demo/RTC Configure/Debouce4 ==
  In1 : Inport  OutDataType=fixdt(1, 16)  OutScaling=2^0
  Add : Sum  Inputs=-+  OutDataTypeMode=int32  OutDataType=fixdt(1, 16)  OutScaling=2^-10  OutDataTypeStr=int32
  Bitwise Operator : simulink/Logic and Bit Operations/Bitwise Operator  logicop=AND  UseBitMask=off  NumInputPorts=2  BitMask=debouce  BitMaskRealWorld=Stored Integer
  Compare To Zero : simulink/Logic and Bit Operations/Compare To Zero  SystemSampleTime=-1  relop===  LogicOutDataTypeMode=uint8  ZeroCross=off
  Compare To Zero1 : simulink/Logic and Bit Operations/Compare To Zero  SystemSampleTime=-1  relop=~=  LogicOutDataTypeMode=boolean  ZeroCross=off
  Constant : Constant  Value=debouce  OutDataTypeMode=int32  OutDataType=fixdt(1, 16)  OutScaling=2^0  OutDataTypeStr=int32
  Constant1 : Constant  Value=mode  OutDataTypeMode=int32  OutDataType=fixdt(1, 16)  OutScaling=2^0  OutDataTypeStr=int32
  Data Type Conversion : DataTypeConversion  OutDataTypeMode=uint32  OutDataType=fixdt(1, 16)  OutScaling=2^0  OutDataTypeStr=uint32
  Enabled Subsystem : Subsystem  TreatAsAtomicUnit=on
  Enabled Subsystem1 : Subsystem  TreatAsAtomicUnit=on
  Enabled Subsystem4 : Subsystem  TreatAsAtomicUnit=on
  Enabled Subsystem5 : Subsystem  TreatAsAtomicUnit=on
  Logical Operator : Logic  AllPortsSameDT=off  OutDataTypeMode=boolean  LogicDataType=fixdt(0, 8)  OutDataTypeStr=boolean
  Logical Operator1 : Logic  Inputs=3  AllPortsSameDT=off  OutDataTypeMode=boolean  LogicDataType=fixdt(0, 8)  OutDataTypeStr=boolean
  Logical Operator{2..3,5,7} (4 alike) : Logic  Operator=NOT  AllPortsSameDT=off  OutDataTypeMode=boolean  LogicDataType=fixdt(0, 8)  OutDataTypeStr=boolean
  Logical Operator4 : Logic  Operator=OR  AllPortsSameDT=off  OutDataTypeMode=boolean  LogicDataType=fixdt(0, 8)  OutDataTypeStr=boolean
  Logical Operator6 : Logic  AllPortsSameDT=off  OutDataTypeMode=boolean  LogicDataType=fixdt(0, 8)  OutDataTypeStr=boolean
  Memory{,1..3} (4 alike) : Memory  LinearizeMemory=on
  Multiport Switch : MultiPortSwitch  OutDataType=fixdt(1, 16)  OutScaling=2^0
  Relational Operator : RelationalOperator  Operator=<  LogicOutDataTypeMode=boolean  LogicDataType=fixdt(0, 8)  OutDataTypeStr=boolean
  Relational Operator1 : RelationalOperator  LogicOutDataTypeMode=boolean  LogicDataType=fixdt(0, 8)  OutDataTypeStr=boolean  InputSameDT=on
  Out1 : Outport  OutDataType=fixdt(1, 16)  OutScaling=2^0
  wires:
  Constant1/1 -> Multiport Switch/1
  Multiport Switch/1 -> Out1/1
  Data Type Conversion/1 -> Bitwise Operator/2
  Enabled Subsystem1/1(Out1) -> Multiport Switch/4
  Logical Operator6/1 -> Enabled Subsystem1/Enable, Multiport Switch/3
  In1/1 -> Compare To Zero/1
  Enabled Subsystem/1(Out1) -> Memory1/1
  Enabled Subsystem4/1(Out1) -> Memory/1
  Memory/1 -> Relational Operator/1, Add/1
  Memory1/1 -> Add/2, Relational Operator/2
  Compare To Zero/1 -> Logical Operator/2, Logical Operator3/1
  Logical Operator/1 -> Enabled Subsystem4/Enable
  Relational Operator/1 -> Logical Operator/1
  Add/1 -> Relational Operator1/1
  Constant/1 -> Data Type Conversion/1, Relational Operator1/2
  Logical Operator2/1 -> Logical Operator1/2
  Memory3/1 -> Logical Operator4/2, Logical Operator5/1
  Logical Operator5/1 -> Logical Operator1/3
  Logical Operator3/1 -> Logical Operator1/1
  Compare To Zero1/1 -> Memory3/1
  Bitwise Operator/1 -> Compare To Zero1/1
  Enabled Subsystem5/1(Out1) -> Bitwise Operator/1
  Logical Operator4/1 -> Enabled Subsystem5/Enable, Memory2/1, Logical Operator6/1
  Memory2/1 -> Logical Operator7/1
  Logical Operator7/1 -> Logical Operator6/2
  Relational Operator1/1 -> Multiport Switch/2, Logical Operator4/1, Logical Operator2/1
  Logical Operator1/1 -> Enabled Subsystem/Enable

== system stm32f4_rtc_configure_demo/RTC Configure/Enabled Subsystem ==
  note: # Mode ID
      | 0 - DD
      | 1 - MM
      | 2 - YY
      | 3 - HH
      | 4 - MM
      | 5 - SS
  UP : Inport  OutDataType=fixdt(1, 16)  OutScaling=2^0
  DOWN : Inport  Port=2  OutDataType=fixdt(1, 16)  OutScaling=2^0
  MODE : Inport  Port=3  OutDataType=fixdt(1, 16)  OutScaling=2^0
  Enable : EnablePort
  Debouce1 : Subsystem  TreatAsAtomicUnit=on  mask{mode=Single Pulse, prescale=4, debouce=4}
      mask prompts: prescale "Prescale (Debouce count)"; debouce "Debouce value"
      settings: RTWFcnNameOpts=Use subsystem name  RTWFileNameOpts=Use function name
      mask StyleString: popup(Normal|Single Pulse|Toggle Latch),popup(4|8|16|32|64|128|256|512|1024|2048|4096|8192),edit
      mask CallbackString: waijung_intput_validation_callback('mode');||waijung_intput_validation_callback('prescale');
      mask Display: disp('Button Pressed\n(Single Pulse)\nDebounce count: 4');
  Debouce2 : Subsystem  TreatAsAtomicUnit=on  mask{mode=Single Pulse, prescale=4, debouce=4}
      mask prompts: prescale "Prescale (Debouce count)"; debouce "Debouce value"
      settings: RTWFcnNameOpts=Use subsystem name  RTWFileNameOpts=Use function name
      mask StyleString: popup(Normal|Single Pulse|Toggle Latch),popup(4|8|16|32|64|128|256|512|1024|2048|4096|8192),edit
      mask CallbackString: waijung_intput_validation_callback('mode');||waijung_intput_validation_callback('prescale');
      mask Display: disp('Button Pressed\n(Single Pulse)\nDebounce count: 4');
  Debouce3 : Subsystem  TreatAsAtomicUnit=on  mask{mode=Single Pulse, prescale=4, debouce=4}
      mask prompts: prescale "Prescale (Debouce count)"; debouce "Debouce value"
      settings: RTWFcnNameOpts=Use subsystem name  RTWFileNameOpts=Use function name
      mask StyleString: popup(Normal|Single Pulse|Toggle Latch),popup(4|8|16|32|64|128|256|512|1024|2048|4096|8192),edit
      mask CallbackString: waijung_intput_validation_callback('mode');||waijung_intput_validation_callback('prescale');
      mask Display: disp('Button Pressed\n(Single Pulse)\nDebounce count: 4');
  Generate Mode ID : Subsystem
  Logical Operator : Logic  Operator=OR  AllPortsSameDT=off  OutDataTypeMode=boolean  LogicDataType=fixdt(0, 8)  OutDataTypeStr=boolean
  Subsystem : Subsystem
  Adjust state : Outport  OutDataType=fixdt(1, 16)  OutScaling=2^0
  wires:
  Logical Operator/1 -> Subsystem/Enable
  Debouce2/1(Out1) -> Subsystem/1(Up), Logical Operator/1
  Debouce3/1(Out1) -> Subsystem/2(Down), Logical Operator/2
  Generate Mode ID/1(Out1) -> Subsystem/3(Adjust State), Adjust state/1
  Debouce1/1(Out1) -> Generate Mode ID/1(In1)
  MODE/1 -> Debouce1/1(In1)
  DOWN/1 -> Debouce3/1(In1)
  UP/1 -> Debouce2/1(In1)

== system stm32f4_rtc_configure_demo/RTC Configure/Debouce4/Enabled Subsystem ==
  Enable : EnablePort
  Counter Free-Running : simulink/Sources/Counter Free-Running  SystemSampleTime=-1  NumBits=32  tsamp=-1
  Out1 : Outport  OutDataType=fixdt(1, 16)  OutScaling=2^0  InitialOutput=0
  wires:
  Counter Free-Running/1 -> Out1/1

== system stm32f4_rtc_configure_demo/RTC Configure/Debouce4/Enabled Subsystem1 ==
  Enable : EnablePort
  Bitwise Operator : simulink/Logic and Bit Operations/Bitwise Operator  logicop=AND  UseBitMask=on  BitMask=1  BitMaskRealWorld=Stored Integer
  Compare To Zero : simulink/Logic and Bit Operations/Compare To Zero  SystemSampleTime=-1  relop===  LogicOutDataTypeMode=uint8  ZeroCross=off
  Counter Free-Running : simulink/Sources/Counter Free-Running  SystemSampleTime=-1  NumBits=32  tsamp=-1
  Out1 : Outport  OutDataType=fixdt(1, 16)  OutScaling=2^0  InitialOutput=0
  wires:
  Counter Free-Running/1 -> Bitwise Operator/1
  Bitwise Operator/1 -> Compare To Zero/1
  Compare To Zero/1 -> Out1/1

== system stm32f4_rtc_configure_demo/RTC Configure/Debouce4/Enabled Subsystem4 ==
  Enable : EnablePort
  Counter Free-Running : simulink/Sources/Counter Free-Running  SystemSampleTime=-1  NumBits=32  tsamp=-1
  Out1 : Outport  OutDataType=fixdt(1, 16)  OutScaling=2^0  InitialOutput=0
  wires:
  Counter Free-Running/1 -> Out1/1

== system stm32f4_rtc_configure_demo/RTC Configure/Debouce4/Enabled Subsystem5 ==
  Enable : EnablePort
  Counter Free-Running : simulink/Sources/Counter Free-Running  SystemSampleTime=-1  NumBits=32  tsamp=-1
  Out1 : Outport  OutDataType=fixdt(1, 16)  OutScaling=2^0  InitialOutput=0
  wires:
  Counter Free-Running/1 -> Out1/1
